simulink model "task_2"  (R2023b)
settings: Solver=FixedStepAuto  StartTime=0.0  StopTime=100  FixedStep=1e-3  RelTol=1e-3
values from neighbouring files (symbols this model uses):
  gamma = 15    [task_1.m]
  lambda = 4    [task_1.m]
  sigma = 0.1    [task_1.m]
  theta = 6    [task_1.m]
  x_init = 1    [task_1.m]
  x_m_init = 2    [task_1.m]
settings Model: Creator=nguye  LastModifiedBy=nguye

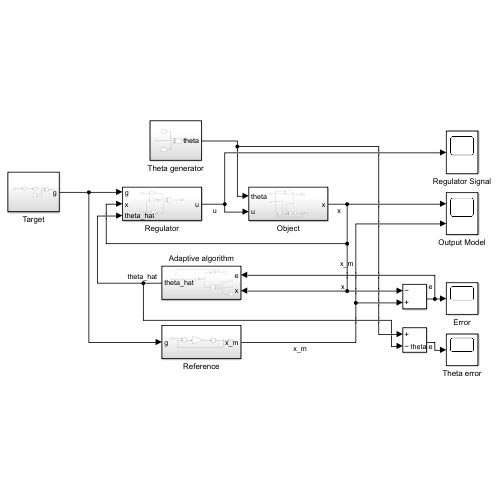
[thumbnail: Simulink's stored preview of the top-level diagram]
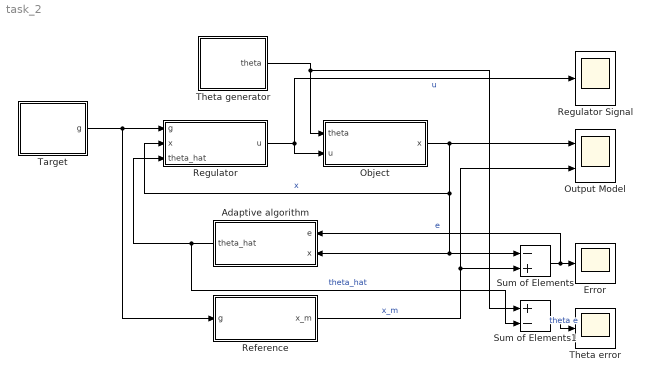
== system task_2 ==
  Adaptive algorithm : Subsystem
  Error : Scope
  Object : Subsystem
  Output Model : Scope  NumInputPorts=2
  Reference : Subsystem
  Regulator : Subsystem
  Regulator Signal : Scope
  Sum of Elements : Sum  Inputs=-+
  Sum of Elements1 : Sum  Inputs=+-
  Target : Subsystem
  Theta error : Scope
  Theta generator : Subsystem
  wires:
  Target/1(g) -> Reference/1(g), Regulator/1(g)
  Regulator/1(u) -> Regulator Signal/1, Object/2(u)  "u"
  Object/1(x) -> Sum of Elements/1, Adaptive algorithm/2(x), Regulator/2(x), Output Model/1  "x"
  Reference/1(x_m) -> Output Model/2, Sum of Elements/2  "x_m"
  Sum of Elements/1 -> Error/1, Adaptive algorithm/1(e)  "e"
  Adaptive algorithm/1(theta_hat) -> Regulator/3(theta_hat), Sum of Elements1/2  "theta_hat"
  Theta generator/1(theta) -> Object/1(theta), Sum of Elements1/1
  Sum of Elements1/1 -> Theta error/1  "theta e"

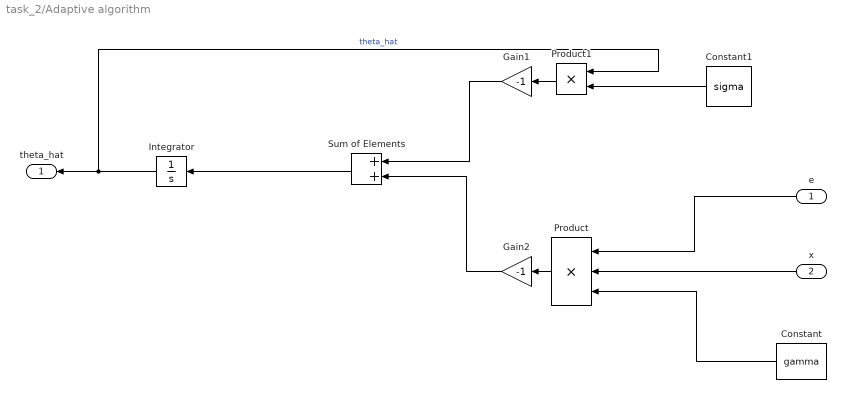
== system task_2/Adaptive algorithm ==
  e : Inport
  x : Inport  Port=2
  Constant : Constant  Value=gamma
  Constant1 : Constant  Value=sigma
  Gain1 : Gain  Gain=-1
  Gain2 : Gain  Gain=-1
  Integrator : Integrator
  Product : Product  Inputs=3
  Product1 : Product
  Sum of Elements : Sum
  theta_hat : Outport
  wires:
  Constant/1 -> Product/3
  e/1 -> Product/1
  x/1 -> Product/2
  Sum of Elements/1 -> Integrator/1
  Integrator/1 -> Product1/1, theta_hat/1  "theta_hat"
  Constant1/1 -> Product1/2
  Product1/1 -> Gain1/1
  Product/1 -> Gain2/1
  Gain1/1 -> Sum of Elements/1
  Gain2/1 -> Sum of Elements/2

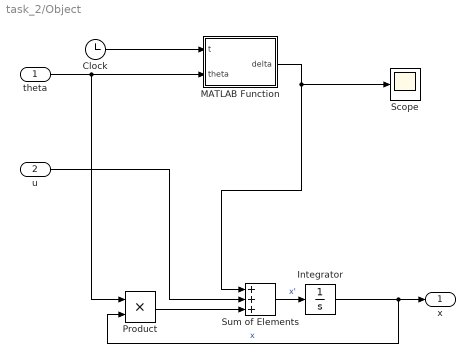
== system task_2/Object ==
  theta : Inport
  u : Inport  Port=2
  Clock : Clock
  Integrator : Integrator  InitialCondition=x_init
  MATLAB Function : MATLAB Function  TreatAsAtomicUnit=on
  Product : Product
  Scope : Scope
  Sum of Elements : Sum  Inputs=+++
  x : Outport
  wires:
  Integrator/1 -> Product/2, x/1  "x"
  Product/1 -> Sum of Elements/3
  Sum of Elements/1 -> Integrator/1  "x'"
  u/1 -> Sum of Elements/2
  Clock/1 -> MATLAB Function/1(t)
  MATLAB Function/1(delta) -> Scope/1, Sum of Elements/1
  theta/1 -> Product/1, MATLAB Function/2(theta)

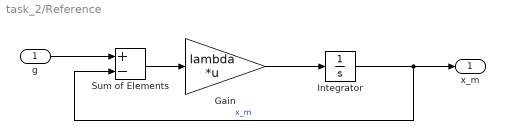
== system task_2/Reference ==
  g : Inport
  Gain : Gain  Gain=lambda  Multiplication=Matrix(K*u)
  Integrator : Integrator  InitialCondition=x_m_init
  Sum of Elements : Sum  Inputs=+-
  x_m : Outport
  wires:
  Gain/1 -> Integrator/1
  Integrator/1 -> Sum of Elements/2, x_m/1  "x_m"
  g/1 -> Sum of Elements/1
  Sum of Elements/1 -> Gain/1

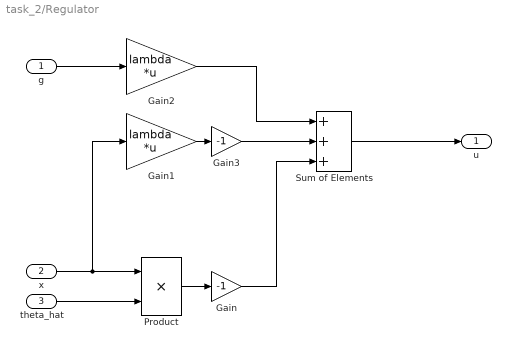
== system task_2/Regulator ==
  g : Inport
  x : Inport  Port=2
  theta_hat : Inport  Port=3
  Gain : Gain  Gain=-1
  Gain1 : Gain  Gain=lambda  Multiplication=Matrix(K*u)
  Gain2 : Gain  Gain=lambda  Multiplication=Matrix(K*u)
  Gain3 : Gain  Gain=-1
  Product : Product
  Sum of Elements : Sum  Inputs=+++
  u : Outport
  wires:
  g/1 -> Gain2/1
  Sum of Elements/1 -> u/1
  Gain2/1 -> Sum of Elements/1
  Gain1/1 -> Gain3/1
  Product/1 -> Gain/1
  x/1 -> Gain1/1, Product/1
  theta_hat/1 -> Product/2
  Gain/1 -> Sum of Elements/3
  Gain3/1 -> Sum of Elements/2

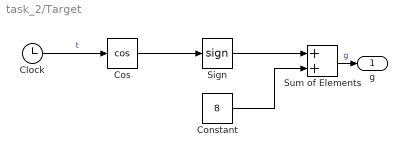
== system task_2/Target ==
  Clock : Clock
  Constant : Constant  Value=8
  Cos : Trigonometry  Operator=cos
  Sign : Signum
  Sum of Elements : Sum
  g : Outport
  wires:
  Clock/1 -> Cos/1  "t"
  Cos/1 -> Sign/1
  Sign/1 -> Sum of Elements/1
  Constant/1 -> Sum of Elements/2
  Sum of Elements/1 -> g/1  "g"

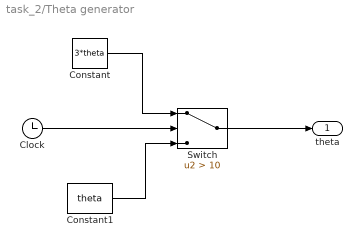
== system task_2/Theta generator ==
  Clock : Clock
  Constant : Constant  Value=3*theta
  Constant1 : Constant  Value=theta
  Switch : Switch  Criteria=u2 > Threshold  Threshold=10  SaturateOnIntegerOverflow=off  InputSameDT=off
  theta : Outport
  wires:
  Clock/1 -> Switch/2
  Constant/1 -> Switch/1
  Constant1/1 -> Switch/3
  Switch/1 -> theta/1

== matlab function task_2/Object/MATLAB Function ==
  data: t input; delta output; theta input
function delta = fcn(t, theta)

p1 = (1+t)^(-1/8);
p2 = 1 - theta*(1+t)^(-1/4) - 3/8*(1+t)^(-5/4);

delta = p1*p2;
